simulink model "TBRe19_ECU_Test_04_Digital_Input"  (R2017b)
settings: Solver=FixedStepDiscrete  StartTime=0.0  StopTime=inf  FixedStep=0.0001  RelTol=1e-3
PostLoadFcn:
  | model_init();
InitFcn:
  | model_check();
PostSaveFcn:
  | model_save();
settings Model: SimulationMode=external  TunableVars=U_BATT_ACTUATEUR_MESURE,ECART_POSITION_ACT_1,ECART_POSITION_ACT_2,CONSIGNE_ACT_1,CONSIGNE_ACT_2,POSITION_ACT_1,POSITION_ACT_2,PAR_FREQ_PWM_ACT_1,PAR_FREQ_MOT_ACT_1,PAR_PROP_MOT_ACT_1,PAR_FREQ_PWM_ACT_2,PAR_FREQ_MOT_ACT_2,PAR_PROP_MOT_ACT_2,PAR_INTRG_MOT_ACT_2  TunableVarsStorageClass=ImportedExtern,ImportedExtern,ImportedExtern,ImportedExtern,ImportedExtern,ImportedExtern,ImportedExtern,ImportedExtern,ImportedExtern,ImportedExtern,ImportedExtern,ImportedExtern,ImportedExtern,ImportedExtern  TunableVarsTypeQualifier=_SAVEDRAM_ , _SAVEDRAM_ , _SAVEDRAM_ , _SAVEDRAM_ , _SAVEDRAM_ , _SAVEDRAM_ , _SAVEDRAM_ , _SAVEDRAM_ , _SAVEDRAM_ , _SAVEDRAM_ , _SAVEDRAM_ , _SAVEDRAM_ , _SAVEDRAM_ , _SAVEDRAM_  Creator=agf25  LastModifiedBy=uvind
settings DataIOCC: LimitDataPoints=on
settings OptimizationCC: DefaultParameterBehavior=Inlined  EfficientFloat2IntCast=on  LifeSpan=inf
settings DebuggingCC: AllowSymbolicDim=off  SFUnexpectedBacktrackingDiag=warning  SFNoUnconditionalDefaultTransitionDiag=warning  SFExecutionAtInitializationDiag=none
settings ModelReferenceCC: PropagateSignalLabelsOutOfModel=off
settings RTWCC: SystemTargetFile=nsi_mpc.tlc  MakeCommand=nsi_make  TemplateMakefile=nsi_mpc.tmf  Description=RTW Coder for MUXLAB4
settings CodeAppCC: StateflowObjectComments=on
settings STFCustomTargetCC: MATLABClassNameForMDSCustomization=Simulink.SoftwareTarget.TargetSpecificTriggerConfigurationBase  SystemTargetFile=nsi_mpc.tlc
settings ConfigComp: CovMetricSettings=dw  CovHtmlReporting=on  CovSaveCumulativeToWorkspaceVar=on  CovSaveSingleToWorkspaceVar=on  CovExternalEMLEnable=off
settings SimscapeCC: SimscapeNormalizeSystem=off
settings ConfigurationSet: Description=SimMechanics 2G

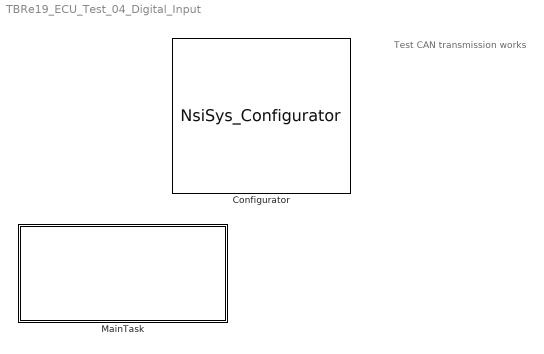
== system TBRe19_ECU_Test_04_Digital_Input ==
  note: Test CAN transmission works
  Configurator : S-Function  FunctionName=NsiSys_Configurator  Parameters=main,io,nbof_can,can,ccp,flash,nbof_lin,lin,tasks  SFunctionDeploymentMode=off  EnableBusSupport=off  mask(Configurator block){main=Config description;01/01/2011;0;0.000000, io=2.5;1;1;1;1;1;1;1;1, nbof_can=5, can=1;HIGH_SPEED;500Kbps;120 Ohm;C:\MUXlink\Install\MUXlink\work\TBRe19_DBC_190621.dbc;0;1;1Mbits;0;HIGH_SPEED;500Kbps;120 Ohm;C:\Users\TBRe-admin\Documents\Database\TBRe19_DBC_190517.dbc;0;0;1Mbits;0;HIGH_SPEED;1000Kbps;120 Ohm;D:\TOOLS\MUXLINK\R2011b\MUXlink\misc\BASE_CAN_MUXLAB4.dbc;0;0;1Mbits;0;HIGH_SPEED;500Kbps;120 Ohm;D:\TOOLS\MUXLINK\R2011b\MUXlink\misc\j1939_adapt.dbc;0;1;1Mbits;0;HIGH_SPEED;1000Kbps;No;D:\TOOLS\MUXLINK\R2011b\MUXlink\misc\BASE_CAN_MUXLAB4.dbc;0;0;1Mbits, ccp=2;0x100;0x200;0;0;0x0;0x0;0;0x13, flash=VAR_NOMBRE_TOT_CYC;No;Unsigned Double Word;0;1;VAR_VBATT_CYC;No;Unsigned Word;12.0;1;VAR_ACT_ACTIF_CYC;No;Unsigned Byte;1;1;VAR_TYP_ACTU_CYC;No;Unsigned Byte;63;1;VAR_MOD_CYC;No;Unsigned Byte;1;1;VAR_SEUIL_COURANT_CYC;No;Unsigned Word;1;1;VAR_ECART_POS_VANNE_CYC;No;Unsigned Byte;1;1;CMPT_NB_CYCLES_REALISE;No;Single Float;0;1;U_BATT_ACTUATEUR_MESURE;Yes;Single Float;0;1;VAR_ETAT_COM_PC;No;Unsigned Byte;0;1;VAR_ETAT_AU;No;Boolean;0;1;VAR_ETAT_MOYEN;No;Unsigned Byte;0;1;VAR_CYCLE_MORPHEE;No;Boolean;0;1;VAR_ETAT_TEST_MORPHEE;No;Boolean;0;1;I_MAX_ATTEINT_ACT_1;No;Boolean;0;1;I_MAX_ATTEINT_ACT_2;No;Boolean;0;1;ECART_POSITION_ACT_1;Yes;Unsigned Byte;0;1;ECART_POSITION_ACT_2;Yes;Unsigned Byte;0;1;DEFAUT_ACT_1;No;Boolean;0;1;DEFAUT_ACT_2;No;Boolean;0;1;CONSIGNE_ACT_1;Yes;Unsigned Byte;0;1;CONSIGNE_ACT_2;Yes;Unsigned Byte;0;1;POSITION_ACT_1;Yes;Unsigned Byte;0;1;POSITION_ACT_2;Yes;Unsigned Byte;0;1;PAR_FREQ_PWM_ACT_1;Yes;Unsigned Word;0;1;PAR_FREQ_MOT_ACT_1;Yes;Unsigned Word;0;1;PAR_PROP_MOT_ACT_1;Yes;Single Float;1;1;PAR_INTRG_MOT_ACT_1;No;Single Float;0;1;PAR_DERIV_MOT_ACT_1;No;Single Float;0;1;PAR_FREQ_PWM_ACT_2;Yes;Unsigned Word;0;1;PAR_FREQ_MOT_ACT_2;Yes;Unsigned Word;0;1;PAR_PROP_MOT_ACT_2;Yes;Single Float;1;1;PAR_INTRG_MOT_ACT_2;Yes;Single Float;0;1;PAR_DERIV_MOT_ACT_2;No;Single Float;0;1;PAR_LEARN_BUTEE_HAUTE_ACT1;No;Unsigned Byte;0;1;PAR_LEARN_BUTEE_BASSE_ACT1;No;Unsigned Byte;0;1;VAR_LEARN_BUTEES_STATUS_ACT1;No;Unsigned Byte;0;1;PAR_LEARN_BUTEE_HAUTE_ACT2;No;Unsigned Byte;0;1;PAR_LEARN_BUTEE_BASSE_ACT2;No;Unsigned Byte;0;1;VAR_LEARN_BUTEES_STATUS_ACT2;No;Unsigned Byte;0;1;CODAGE_carte0;No;Boolean;0;1;CODAGE_carte1;No;Boolean;0;1, nbof_lin=2, lin=0;D:\TOOLS\MUXLINK\R2011b\MUXlink\misc\lindb.ldf;1;0.0;0.0;0.000;0.000;0.000000;0,0;0;D:\TOOLS\MUXLINK\R2011b\MUXlink\misc\lindb.ldf;1;0.0;0.0;0.000;0.000;0.000000;0,0, tasks=MainTask;[0.01]}
      mask prompts: nbof_can "nbof can"
      mask help: This block permits to set general parameters to use a MUXlink model
      mask init:
      | NsiSys_Configurator_InitializationFcn();
      settings: OpenFcn=NsiSys_Configurator_OpenFcn();
      mask Help:
      | eval('block=get_param(gcb, ''RTWdata'');')
      | web([docroot '\toolbox\MUXlink\html\blocks/' block.MUXlink_BlockType '.html'])
      mask Callback main: NsiSys_Configurator_ApplyFcn(1);
      mask Callback io: NsiSys_Configurator_ApplyFcn(2);
      mask Callback nbof_can: NsiSys_Configurator_ApplyFcn(3);
      mask Callback can: NsiSys_Configurator_ApplyFcn(4);
      mask Callback ccp: NsiSys_Configurator_ApplyFcn(5);
      mask Callback flash: NsiSys_Configurator_ApplyFcn(6);
      mask Callback nbof_lin: NsiSys_Configurator_ApplyFcn(7);
      mask Callback lin: NsiSys_Configurator_ApplyFcn(8);
      mask Callback tasks: NsiSys_Configurator_ApplyFcn(9);
      mask Display: image(imread('MUXLAB4.bmp'));text(0.5, 0.2, '', 'horizontalAlignment', 'center', 'verticalAlignment', 'base');
  MainTask : Subsystem  TreatAsAtomicUnit=on  SystemSampleTime=[0.01]  RTWFcnName=MainTask  RTWFileName=FileTaskFcn
      mask init:
      | NsiSys_SubSystemTask_InitializationFcn();
      settings: OpenFcn=NsiSys_SubSystemTask_OpenFcn();  RTWSystemCode=Nonreusable function  RTWFcnNameOpts=User specified  RTWFileNameOpts=Use function name
      mask Display: image(imread('nsi.bmp'));text(0.45, 0.9, 'task()');plot([0.05 0.05 0.05 0.05 0.05 0.05 0.05 0.05 0.05 0.05]);fprintf('MainTask\n/ 10.0ms / 0.0ms /\nEvent');

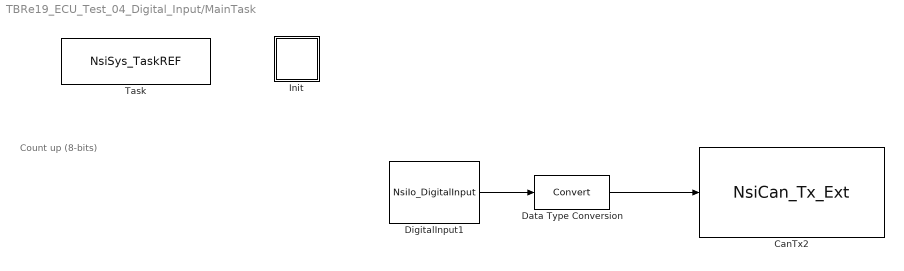
== system TBRe19_ECU_Test_04_Digital_Input/MainTask ==
  note: Count up (8-bits)
  CanTx2 : S-Function  FunctionName=NsiCan_Tx_Ext  Parameters=data_can,channel,msg_name,ident,ident_type,dlc,signals,is_physical,is_canfd,is_crc  SFunctionDeploymentMode=off  EnableBusSupport=off  mask(MUXlink Can Tx){data_can=1;HIGH_SPEED;500Kbps;120 Ohm;C:\MUXlink\Install\MUXlink\work\TBRe19_DBC_190621.dbc;0;;;0;HIGH_SPEED;500Kbps;120 Ohm;C:\Users\TBRe-admin\Documents\Database\TBRe19_DBC_190517.dbc;0;;;0;HIGH_SPEED;1000Kbps;120 Ohm;D:\TOOLS\MUXLINK\R2011b\MUXlink\misc\BASE_CAN_MUXLAB4.dbc;0;;;0;HIGH_SPEED;500Kbps;120 Ohm;D:\TOOLS\MUXLINK\R2011b\MUXlink\misc\j1939_adapt.dbc;0;;;0;HIGH_SPEED;1000Kbps;No;D:\TOOLS\MUXLINK\R2011b\MUXlink\misc\BASE_CAN_MUXLAB4.dbc;0;;, channel=1, msg_name=SteeringWheelSensor, ident=0x234, ident_type=STD, dlc=5, signals=Acc_Angle;1;0;-16;0.100000;0.000000;Degrees, is_physical=0, is_canfd=0, is_crc=0}
      mask prompts: data_can "data can"; msg_name "msg name"
      mask help: Transmit a frame on a CAN Channel.
      mask init:
      | NsiCan_Tx_Ext_InitializationFcn();
      settings: OpenFcn=NsiCan_Tx_Ext_OpenFcn();
      mask Help:
      | eval('block=get_param(gcb, ''RTWdata'');')
      | web([docroot '\toolbox\MUXlink\html\blocks/' block.MUXlink_BlockType '.html'])
      mask Callback data_can: NsiCan_Tx_Ext_ApplyFcn(1);
      mask Callback channel: NsiCan_Tx_Ext_ApplyFcn(2);
      mask Callback msg_name: NsiCan_Tx_Ext_ApplyFcn(3);
      mask Callback ident: NsiCan_Tx_Ext_ApplyFcn(4);
      mask Callback ident_type: NsiCan_Tx_Ext_ApplyFcn(5);
      mask Callback dlc: NsiCan_Tx_Ext_ApplyFcn(6);
      mask Callback signals: NsiCan_Tx_Ext_ApplyFcn(7);
      mask Callback is_physical: NsiCan_Tx_Ext_ApplyFcn(7);
      mask Callback is_canfd: NsiCan_Tx_Ext_ApplyFcn(7);
      mask Callback is_crc: NsiCan_Tx_Ext_ApplyFcn(7);
      mask Display: image(imread('nsi.bmp'));text(0.5, 0.1, 'TX_SteeringWheelSensor_CAN1', 'horizontalAlignment', 'center', 'verticalAlignment', 'base');plot([0.05 0.05 0.05 0.05 0.05 0.05 0.05 0.05 0.05 0.05]); port_label('input',1, 'Acc_Angle');
  Data Type Conversion : DataTypeConversion
  DigitalInput1 : S-Function  FunctionName=NsiIo_DigitalInput  Parameters=channel,is_trigger,typeof_trigger,is_wakeup,wakeup_level  SFunctionDeploymentMode=off  EnableBusSupport=off  mask(MUXlink I/O Digital Input){channel=11, is_trigger=off, typeof_trigger=Either, is_wakeup=off, wakeup_level=Low level}
      mask prompts: channel "Channel ?"; is_trigger "Trigger ?"; typeof_trigger "Type of Trigger ?"; is_wakeup "Wake-up ?"; wakeup_level "Wake-up level ?"
      mask help: Read digital input from I/O channel.
      mask init:
      | NsiIo_DigitalInput_InitializationFcn();
      settings: OpenFcn=NsiIo_DigitalInput_OpenFcn();
      mask Help:
      | eval('block=get_param(gcb, ''RTWdata'');')
      | web([docroot '\toolbox\MUXlink\html\blocks/' block.MUXlink_BlockType '.html'])
      mask Callback channel: NsiIo_DigitalInput_ApplyFcn(1);
      mask Callback is_trigger: NsiIo_DigitalInput_ApplyFcn(2);
      mask TypeOptions typeof_trigger: Rising | Falling | Either
      mask Callback typeof_trigger: NsiIo_DigitalInput_ApplyFcn(3);
      mask Callback is_wakeup: NsiIo_DigitalInput_ApplyFcn(4);
      mask TypeOptions wakeup_level: Low level | High level
      mask Callback wakeup_level: NsiIo_DigitalInput_ApplyFcn(5);
      mask Display: image(imread('nsi.bmp'));text(0.5, 0.2, 'DigitalInput_11', 'horizontalAlignment', 'center', 'verticalAlignment', 'base');plot([0.05 0.05 0.05 0.05 0.05 0.05 0.05 0.05 0.05 0.05]);port_label('output', 1, 'Ground : G1');
  Init : Subsystem  mask(System Initialize){}
      mask help: Add code to a systems Initialize function
      settings: CopyFcn=cccopyfcn(gcb)  OpenFcn=ccopenfcn('System Initialize Function')
      mask Help: This block contains text fields to insert custom user code sections at the declaration, execution and exit sections of the systems initialize function.  By placing this block inside a subsytem, the custom user code will appear in that subsystems function.
      mask Display: disp('I()')
  Task : S-Function  FunctionName=NsiSys_TaskREF  Parameters=task_initialised,task_periodic, task_sampletime,task_name,task_event,task_offset  SFunctionDeploymentMode=off  EnableBusSupport=off  mask(task definition){task_initialised=on, task_periodic=on, task_sampletime=[0.01], task_offset=0.00, task_name=MainTask, task_event=on}
      mask prompts: task_initialised "task initialised"; task_periodic "Is Periodic"; task_sampletime "Task sample time"; task_offset "Task Offset"; task_name "Task name"; task_event "Is event"
      mask help:
      | Permit to provide all parameters associated to a MUXLINK task.
      | Task can be executed periodicaly and/or on event detection.
      | If task is periodic:
      | Task sample time specify the execution period in mS [0.001   6000]
      | Task Offset specify the offset applied to the execution period
      | Task Offset < Task sample time
      mask init:
      | NsiSys_TaskREF_InitializationFcn();
      settings: OpenFcn=NsiSys_Task_OpenFcn();
      mask Callback task_initialised: NsiSys_TaskREF_ApplyFcn(1);
      mask Callback task_periodic: NsiSys_TaskREF_ApplyFcn(2);
      mask Callback task_sampletime: NsiSys_TaskREF_ApplyFcn(3);
      mask Callback task_offset: NsiSys_TaskREF_ApplyFcn(6);
      mask Callback task_name: NsiSys_TaskREF_ApplyFcn(4);
      mask Callback task_event: NsiSys_TaskREF_ApplyFcn(5);
      mask Display: text(0.5, 0.8, 't()', 'horizontalAlignment', 'center', 'verticalAlignment', 'base');text(0.5, 0.2, '/ 10.0ms / 0.0ms /', 'horizontalAlignment', 'center', 'verticalAlignment', 'base');text(0.5, 0.4, 'Event', 'horizontalAlignment', 'center', 'verticalAlignment', 'base');
  wires:
  Data Type Conversion/1 -> CanTx2/1
  DigitalInput1/1 -> Data Type Conversion/1

== system TBRe19_ECU_Test_04_Digital_Input/MainTask/Init ==
